simulink model "lateral_perturbation"  (Simulink 7.4)
settings: Solver=ode45  StartTime=0.0  StopTime=240  FixedStep=0.0033  RelTol=0.0033
libraries: dsparch4 x1, commnoisgen2 x1
settings Model: Creator=Sandy  LastModifiedBy=Sandy
settings SolverCC: ConsecutiveZCsStepRelTol=0.0033
settings DebuggingCC: SolverPrmCheckMsg=none

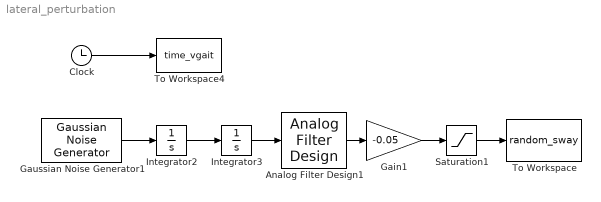
== system lateral_perturbation ==
  Analog Filter Design1 : dsparch4/Analog Filter Design  method=Butterworth  filttype=Highpass  N=2  Wlo=1.3  Whi=80  Rp=2  Rs=40
  Clock : Clock
      settings: Decimation=10
  Gain1 : Gain  Gain=-0.05  ParameterDataType=fixdt(1, 16)  ParameterScaling=2^0  OutDataType=fixdt(1, 16)  OutScaling=2^0
  Gaussian Noise Generator1 : commnoisgen2/Gaussian Noise Generator  SystemSampleTime=-1  m=0  d=200  s=461  Ts=0.0033  frameBased=off  sampPerFrame=1  orient=off  outDataType=double
  Integrator2 : Integrator
  Integrator3 : Integrator
  Saturation1 : Saturate  UpperLimit=0.05  LowerLimit=-0.05  SampleTime=0.0033  OutDataType=fixdt(1, 16)  OutScaling=2^0
  To Workspace : ToWorkspace  VariableName=random_sway  SampleTime=0.0033  SaveFormat=Array
  To Workspace4 : ToWorkspace  VariableName=time_vgait  SampleTime=0.0033  SaveFormat=Array
  wires:
  Clock/1 -> To Workspace4/1
  Integrator2/1 -> Integrator3/1
  Integrator3/1 -> Analog Filter Design1/1
  Saturation1/1 -> To Workspace/1
  Analog Filter Design1/1 -> Gain1/1
  Gain1/1 -> Saturation1/1
  Gaussian Noise Generator1/1 -> Integrator2/1
